simulink model "E3"  (R2016b)
settings: Solver=ode45  StartTime=0.0  StopTime=2  RelTol=1e-3
libraries: simulink x1
settings Model: Creator=jonathankirchman  LastModifiedBy=jonathankirchman

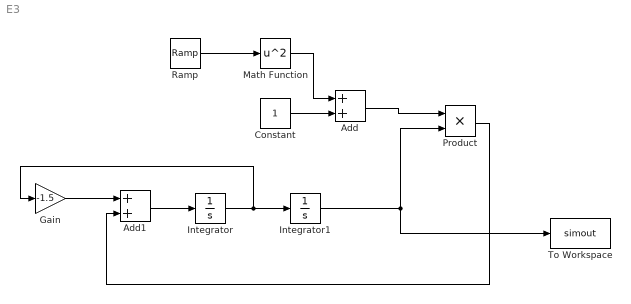
== system E3 ==
  Add : Sum
  Add1 : Sum
  Constant : Constant
  Gain : Gain  Gain=-1.5
  Integrator : Integrator  InitialCondition=0.5
  Integrator1 : Integrator
  Math Function : Math  Operator=square  SaturateOnIntegerOverflow=on
  Product : Product
  Ramp : simulink/Sources/Ramp  slope=1  start=0  X0=0
  To Workspace : ToWorkspace  VariableName=simout  SampleTime=-1
  wires:
  Ramp/1 -> Math Function/1
  Math Function/1 -> Add/1
  Constant/1 -> Add/2
  Add/1 -> Product/1
  Gain/1 -> Add1/1
  Product/1 -> Add1/2
  Add1/1 -> Integrator/1
  Integrator/1 -> Gain/1, Integrator1/1
  Integrator1/1 -> To Workspace/1, Product/2
